simulink model "s8_11"  (Simulink 6.6)
settings: Solver=ode23  SolverMode=SingleTasking  StartTime=0.0  StopTime=t_d  MaxStep=Tc  RelTol=1e-8  AbsTol=1e-8
values from neighbouring files (symbols this model uses):
  F_e = K_r*k_t*inv(R_a)*k_v*K_r    [i8_11.m]
  F_v = K_r*diag([0.01 0.01])*K_r    [i8_11.m]
  g = 9.81    [i8_11.m]
  G_r = K_r*k_t*inv(R_a)*G_v    [i8_11.m]
  k_fa = K_r*k_v*inv(K_v)    [i8_11.m]
  k_fp = k_tp    [i8_11.m]
  k_fv = k_tv    [i8_11.m]
  K_p = 6.25*diag([1 1])    [i8_11.m]
  K_pr = R_a*inv(k_t*K_r)    [i8_11.m]
  k_tp = K_r*k_tp    [i8_11.m]
  k_tv = K_r*k_tv    [i8_11.m]
  K_v = 32*diag([1 1])    [i8_11.m]
  Tc = 0.001    [i8_11.m]
  Ts = Tc    (= 0.001)    [i8_11.m]
undefined symbols (not defined in the file or in its folder): a, Ad, Bd, Cd, Dd, iner_l, pi_l, pi_m, q_i
settings Model: Creator=luigivillani  LastModifiedBy=luigivillani  ExtModeAutoUpdateStatusClock=off
settings SolverCC: InitialStep=0.1*Tc
settings DataIOCC: LimitDataPoints=off  SaveOutput=off  SaveTime=off
settings OptimizationCC: BlockReduction=off  BooleanDataType=off
settings DebuggingCC: SignalResolutionControl=TryResolveAllWithWarning  SolverPrmCheckMsg=none  MultiTaskDSMMsg=warning  MultiTaskCondExecSysMsg=none  StrictBusMsg=None
settings HardwareCC: TargetUnknown=on
settings RTWCC: IncludeERTFirstTime=on

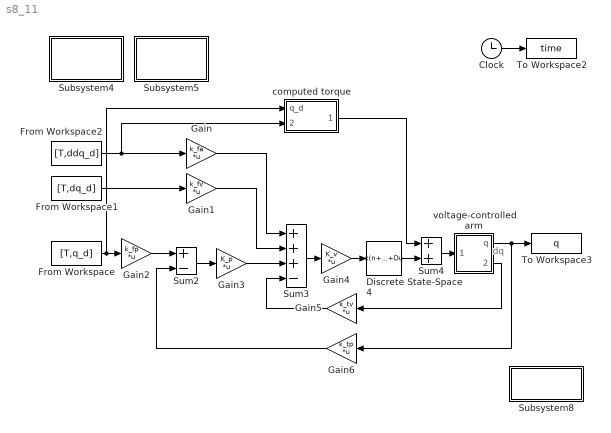
== system s8_11 ==
  note: dq
  Clock : Clock
      settings: Decimation=10
  Discrete State-Space4 : DiscreteStateSpace  A=Ad  B=Bd  C=Cd  D=Dd  X0=[0 0]  SampleTime=Tc
      mask Display: disp('PI')
  From Workspace : FromWorkspace  VariableName=[T,q_d]  SampleTime=Tc
  From Workspace1 : FromWorkspace  VariableName=[T,dq_d]  SampleTime=Tc
  From Workspace2 : FromWorkspace  VariableName=[T,ddq_d]  SampleTime=Tc
  Gain : Gain  Gain=k_fa  Multiplication=Matrix(K*u)  SampleTime=Tc
      mask Display: disp('k_fa')
  Gain1 : Gain  Gain=k_fv  Multiplication=Matrix(K*u)  SampleTime=Tc
      mask Display: disp('k_fv')
  Gain2 : Gain  Gain=k_fp  Multiplication=Matrix(K*u)  SampleTime=Tc
      mask Display: disp('k_fp')
  Gain3 : Gain  Gain=K_p  Multiplication=Matrix(K*u)  SampleTime=Tc
      mask Display: disp('K_p')
  Gain4 : Gain  Gain=K_v  Multiplication=Matrix(K*u)  SampleTime=Tc
      mask Display: disp('K_v')
  Gain5 : Gain  Orientation=left  Gain=k_tv  Multiplication=Matrix(K*u)  SampleTime=Tc
      mask Display: disp('k_tv')
  Gain6 : Gain  Orientation=left  Gain=k_tp  Multiplication=Matrix(K*u)  SampleTime=Tc
      mask Display: disp('k_tp')
  Subsystem4 : Subsystem
      settings: OpenFcn=clear all;c=0;i8_11;
      mask Display: disp('K_p = 5\nK_v = 10')
  Subsystem5 : Subsystem
      settings: OpenFcn=clear all;c=1;i8_11;
      mask Display: disp('K_p = 6.25\nK_v = 32')
  Subsystem8 : Subsystem  Orientation=left
      settings: OpenFcn=p8_11;
      mask Display: disp('plot')
  Sum2 : Sum  Inputs=+-  SaturateOnIntegerOverflow=on  InputSameDT=on
  Sum3 : Sum  Inputs=+++-  SaturateOnIntegerOverflow=on  InputSameDT=on
  Sum4 : Sum  SaturateOnIntegerOverflow=on  InputSameDT=on
  To Workspace2 : ToWorkspace  VariableName=time  SampleTime=Ts  SaveFormat=Array
      settings: MaxDataPoints=5001
  To Workspace3 : ToWorkspace  VariableName=q  SampleTime=Ts  SaveFormat=Array
      settings: MaxDataPoints=5001
  computed torque : Subsystem
      mask Display: disp('tau_d')
  voltage-controlled arm : Subsystem
      mask Display: disp('M')
  wires:
  Sum2/1 -> Gain3/1
  Gain2/1 -> Sum2/1
  Clock/1 -> To Workspace2/1
  From Workspace1/1 -> Gain1/1
  Gain6/1 -> Sum2/2
  voltage-controlled arm/2(dq) -> Gain5/1
  From Workspace/1 -> computed torque/1(q_d), Gain2/1
  From Workspace2/1 -> computed torque/2(dq_d), Gain/1
  Sum4/1 -> voltage-controlled arm/1(Vc)
  Discrete State-Space4/1 -> Sum4/2
  Gain5/1 -> Sum3/4
  Gain1/1 -> Sum3/2
  computed torque/1(tau_d) -> Sum4/1
  Gain4/1 -> Discrete State-Space4/1
  Sum3/1 -> Gain4/1
  voltage-controlled arm/1(q) -> To Workspace3/1, Gain6/1
  Gain/1 -> Sum3/1
  Gain3/1 -> Sum3/3

== system s8_11/Subsystem4 ==
  note: start

== system s8_11/Subsystem5 ==
  note: start

== system s8_11/Subsystem8 ==
  note: start

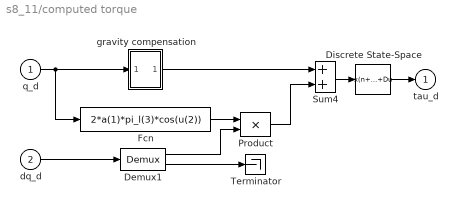
== system s8_11/computed torque ==
  q_d : Inport
  dq_d : Inport  Port=2
  Demux1 : Demux  Outputs=2
  Discrete State-Space : DiscreteStateSpace  A=0  B=zeros(1,2)  C=zeros(2,1)  D=K_pr  SampleTime=Tc
      mask Display: disp('K_pr')
  Fcn : Fcn  Expr=2*a(1)*pi_l(3)*cos(u(2))
  Product : Product  SaturateOnIntegerOverflow=on  RndMeth=Zero  InputSameDT=on
  Sum4 : Sum  SaturateOnIntegerOverflow=on  InputSameDT=on
  Terminator : Terminator
  gravity compensation : Subsystem
      mask Display: disp('g(q)')
  tau_d : Outport  InitialOutput=0
  wires:
  Discrete State-Space/1 -> tau_d/1
  dq_d/1 -> Demux1/1
  Fcn/1 -> Product/1
  Demux1/1 -> Product/2
  gravity compensation/1(out_1) -> Sum4/1
  Product/1 -> Sum4/2
  Sum4/1 -> Discrete State-Space/1
  q_d/1 -> gravity compensation/1(in_1), Fcn/1
  Demux1/2 -> Terminator/1

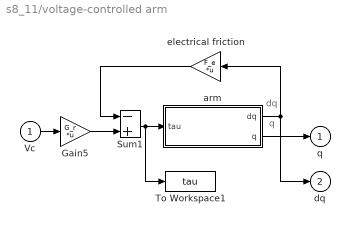
== system s8_11/voltage-controlled arm ==
  note: dq
  note: q
  Vc : Inport
  Gain5 : Gain  Gain=G_r  Multiplication=Matrix(K*u)  SampleTime=0
      mask Display: disp('G_r')
  Sum1 : Sum  Inputs=-+  SaturateOnIntegerOverflow=on  InputSameDT=on
  To Workspace1 : ToWorkspace  VariableName=tau  SampleTime=Ts  SaveFormat=Array
      settings: MaxDataPoints=5001
  arm : Subsystem
      mask Display: disp('inv(B(q))(tau-tau'')')
  electrical friction : Gain  Orientation=left  Gain=F_e  Multiplication=Matrix(K*u)  SampleTime=0
      mask Display: disp('F_e')
  q : Outport  InitialOutput=0
  dq : Outport  Port=2  InitialOutput=0
  wires:
  Vc/1 -> Gain5/1
  Gain5/1 -> Sum1/2
  electrical friction/1 -> Sum1/1
  arm/2("q ") -> q/1
  arm/1(dq) -> dq/1, electrical friction/1
  Sum1/1 -> To Workspace1/1, arm/1(tau)

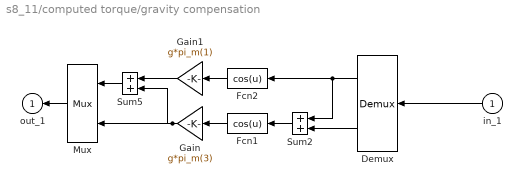
== system s8_11/computed torque/gravity compensation ==
  in_1 : Inport  Orientation=left
  Demux : Demux  Orientation=left  Outputs=2
  Fcn1 : Fcn  Orientation=left  Expr=cos(u)
  Fcn2 : Fcn  Orientation=left  Expr=cos(u)
  Gain : Gain  Orientation=left  Gain=g*pi_m(3)  SaturateOnIntegerOverflow=on
      mask Display: disp('k_2')
  Gain1 : Gain  Orientation=left  Gain=g*pi_m(1)  SaturateOnIntegerOverflow=on
      mask Display: disp('k_1')
  Mux : Mux  Orientation=left  Inputs=2
  Sum2 : Sum  Orientation=left  SaturateOnIntegerOverflow=on  InputSameDT=on
  Sum5 : Sum  Orientation=left  SaturateOnIntegerOverflow=on  InputSameDT=on
  out_1 : Outport  Orientation=left  InitialOutput=0
  wires:
  in_1/1 -> Demux/1
  Demux/2 -> Sum2/2
  Sum2/1 -> Fcn1/1
  Fcn1/1 -> Gain/1
  Fcn2/1 -> Gain1/1
  Demux/1 -> Fcn2/1, Sum2/1
  Gain1/1 -> Sum5/1
  Sum5/1 -> Mux/1
  Gain/1 -> Mux/2, Sum5/2
  Mux/1 -> out_1/1

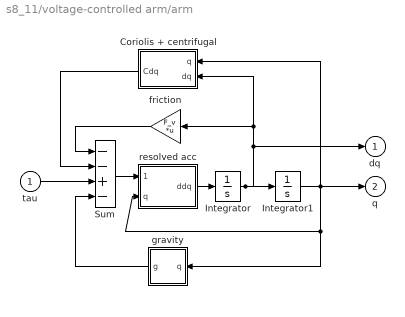
== system s8_11/voltage-controlled arm/arm ==
  tau : Inport
  Coriolis + centrifugal : Subsystem  Orientation=left
      mask Display: disp('C(q,dq)dq')
  Integrator : Integrator  InitialCondition=[0 0]  ZeroCross=off
  Integrator1 : Integrator  InitialCondition=q_i  ZeroCross=off
  Sum : Sum  Inputs=--+-  SaturateOnIntegerOverflow=on  InputSameDT=on
  friction : Gain  Orientation=left  Gain=F_v  Multiplication=Matrix(K*u)  SaturateOnIntegerOverflow=on
      mask Display: disp('F_v')
  gravity : Subsystem  Orientation=left
      mask Display: disp('g(q)')
  resolved acc : Subsystem
      mask Display: disp('inv(B(q))')
  dq : Outport  InitialOutput=0
  "q " : Outport  Port=2  InitialOutput=0
  wires:
  Coriolis + centrifugal/1(Cdq) -> Sum/2
  tau/1 -> Sum/3
  Integrator1/1 -> Coriolis + centrifugal/1(q), resolved acc/2(q), gravity/1(q), "q "/1
  resolved acc/1(ddq) -> Integrator/1
  Integrator/1 -> Integrator1/1, dq/1, Coriolis + centrifugal/2(dq), friction/1
  Sum/1 -> resolved acc/1(tau-tau')
  friction/1 -> Sum/1
  gravity/1(g) -> Sum/4

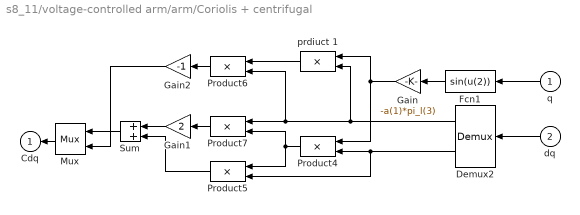
== system s8_11/voltage-controlled arm/arm/Coriolis + centrifugal ==
  q : Inport  Orientation=left
  dq : Inport  Orientation=left  Port=2
  Demux2 : Demux  Orientation=left  Outputs=2
  Fcn1 : Fcn  Orientation=left  Expr=sin(u(2))
  Gain : Gain  Orientation=left  Gain=-a(1)*pi_l(3)  SaturateOnIntegerOverflow=on
      mask Display: disp('k_3')
  Gain1 : Gain  Orientation=left  Gain=2  SaturateOnIntegerOverflow=on
  Gain2 : Gain  Orientation=left  Gain=-1  SaturateOnIntegerOverflow=on
  Mux : Mux  Orientation=left  Inputs=2
  Product{4..7} (4 alike) : Product  Orientation=left  SaturateOnIntegerOverflow=on  RndMeth=Zero  InputSameDT=on
  Sum : Sum  Orientation=left  SaturateOnIntegerOverflow=on  InputSameDT=on
  prdiuct 1 : Product  Orientation=left  SaturateOnIntegerOverflow=on  RndMeth=Zero  InputSameDT=on
  Cdq : Outport  Orientation=left  InitialOutput=0
  wires:
  dq/1 -> Demux2/1
  Gain2/1 -> Mux/2
  Product6/1 -> Gain2/1
  Mux/1 -> Cdq/1
  Sum/1 -> Mux/1
  Product5/1 -> Sum/2
  Gain1/1 -> Sum/1
  Product7/1 -> Gain1/1
  Demux2/1 -> prdiuct 1/2, Product6/2, Product7/1
  Demux2/2 -> Product4/2, Product5/2
  prdiuct 1/1 -> Product6/1
  Gain/1 -> prdiuct 1/1, Product4/1
  Fcn1/1 -> Gain/1
  q/1 -> Fcn1/1
  Product4/1 -> Product5/1, Product7/2

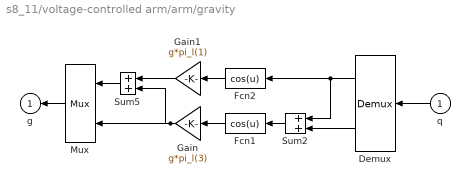
== system s8_11/voltage-controlled arm/arm/gravity ==
  q : Inport  Orientation=left
  Demux : Demux  Orientation=left  Outputs=2
  Fcn1 : Fcn  Orientation=left  Expr=cos(u)
  Fcn2 : Fcn  Orientation=left  Expr=cos(u)
  Gain : Gain  Orientation=left  Gain=g*pi_l(3)  SaturateOnIntegerOverflow=on
      mask Display: disp('k_2')
  Gain1 : Gain  Orientation=left  Gain=g*pi_l(1)  SaturateOnIntegerOverflow=on
      mask Display: disp('k_1')
  Mux : Mux  Orientation=left  Inputs=2
  Sum2 : Sum  Orientation=left  SaturateOnIntegerOverflow=on  InputSameDT=on
  Sum5 : Sum  Orientation=left  SaturateOnIntegerOverflow=on  InputSameDT=on
  g : Outport  Orientation=left  InitialOutput=0
  wires:
  q/1 -> Demux/1
  Demux/2 -> Sum2/2
  Sum2/1 -> Fcn1/1
  Fcn1/1 -> Gain/1
  Fcn2/1 -> Gain1/1
  Demux/1 -> Fcn2/1, Sum2/1
  Gain1/1 -> Sum5/1
  Sum5/1 -> Mux/1
  Gain/1 -> Sum5/2, Mux/2
  Mux/1 -> g/1

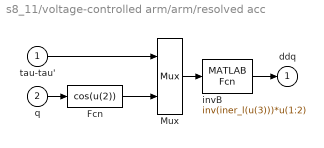
== system s8_11/voltage-controlled arm/arm/resolved acc ==
  tau-tau' : Inport
  q : Inport  Port=2
  Fcn : Fcn  Expr=cos(u(2))
  Mux : Mux  Inputs=[2,1]
  "invB " : MATLABFcn  MATLABFcn=inv(iner_l(u(3)))*u(1:2)  OutputDimensions=2
      mask Display: disp('inv(B(q))')
  ddq : Outport  InitialOutput=0
  wires:
  Fcn/1 -> Mux/2
  q/1 -> Fcn/1
  "invB "/1 -> ddq/1
  tau-tau'/1 -> Mux/1
  Mux/1 -> "invB "/1
